simulink model "final4dof"  (R2016b)
settings: Solver=VariableStepAuto  StartTime=0.0  StopTime=inf  RelTol=1e-3
StartFcn:
  | 1
values from neighbouring files (symbols this model uses):
  N = sqrt(1-M*M)    [GUI_TA.m]
undefined symbols (not defined in the file or in its folder): final4dof, RootGround, RootPart
libraries: mblibv1 x18, simulink x4
settings Model: Creator=IMA F  LastModifiedBy=MILZAM_WAFI
settings OptimizationCC: BlockReduction=off
settings SimMechanicsCC: VisOnUpdateDiagram=on  VisDuringSimulation=on

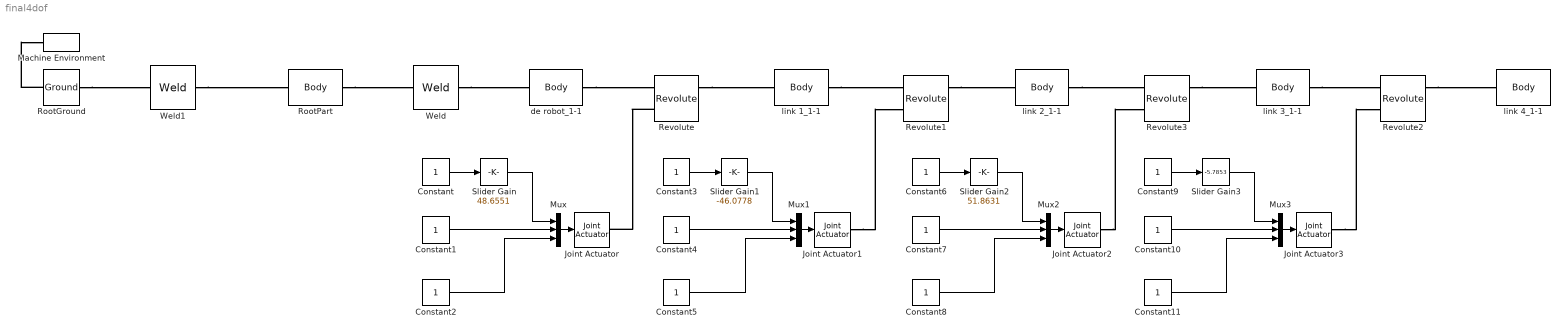
== system final4dof ==
  Constant{,1..11} (12 alike) : Constant
  Joint Actuator{,1..3} (4 alike) : mblibv1/Sensors &  Actuators/Joint Actuator  UpdateFromCAD=off  PhysicalDomain=Mechanical  PortType=blob  ActuationStyle=Motion  AngleUnits=deg  ArcVelocityUnits=deg/s  ArcAccelerationUnits=deg/s^2  CoordPositionUnits=m  VelocityUnits=m/s  AccelerationUnits=m/s^2  ForceUnits=N  TorqueUnits=N*m  ActiveIO=on  Width=3  DialogClass=MechanicalActuatorBlock  Primitive=R1  ReferenceFrame=Absolute (World)
  Machine Environment : mblibv1/Bodies/Machine Environment  PortType=env  PhysicalDomain=Mechanical  DialogTemplateClass=MECH.MachineEnvironment  SyncWhenCopied=off  Gravity=[0 -9.81 0]  GravityUnits=m/s^2  GravityAsSignal=off  Dimensionality=Auto-detect  AnalysisType=Forward dynamics  LinearAssemblyTolerance=1e-3  LinearAssemblyToleranceUnits=m  AngularAssemblyTolerance=1e-3  AngularAssemblyToleranceUnits=rad  ConstraintSolverType=Stabilizing  ConstraintRelTolerance=1e-4  ConstraintAbsTolerance=1e-4  UseRobustSingularityHandling=off  RedundancyAnalysisToleranceType=Automatically select tolerance  RedundancyAnalysisTolerance=1e-14  StatePerturbationType=Fixed  PerturbationSize=1e-5  VisualizeMachine=on  BodyVisualizationType=Use model default body geometries  BodyColorSelMode=Use model default  DefaultBodyColor=[1 0 0]
  Mux{,1..3} (4 alike) : Mux  Inputs=3
  Revolute : mblibv1/Joints/Revolute  LConnTagsString=__newl0|SA1  RConnTagsString=__newr0|SA1  UpdateFromCAD=on  PMImportedID=de robot_1-1:-:link 1_1-1  NumSAPorts=2  CutJoint=off  MarkAsCut=off  Primitives=prismatic  PrimitiveProps=R1$World$[0,0,-1]$revolute  DialogClass=JointBlock  R1Axis=[0,0,-1]
  Revolute1 : mblibv1/Joints/Revolute  LConnTagsString=__newl0|SA1  RConnTagsString=__newr0|SA1  UpdateFromCAD=on  PMImportedID=link 1_1-1:-:link 2_1-1  NumSAPorts=2  CutJoint=off  MarkAsCut=off  Primitives=prismatic  PrimitiveProps=R1$World$[-0.659109,-0.752048,0]$revolute  DialogClass=JointBlock  R1Axis=[-0.659109,-0.752048,0]
  Revolute2 : mblibv1/Joints/Revolute  LConnTagsString=__newl0|SA1  RConnTagsString=__newr0|SA1  UpdateFromCAD=on  PMImportedID=link 3_1-1:-:link 4_1-1  NumSAPorts=2  CutJoint=off  MarkAsCut=off  Primitives=prismatic  PrimitiveProps=R1$World$[-0.659109,-0.752048,0]$revolute  DialogClass=JointBlock  R1Axis=[-0.659109,-0.752048,0]
  Revolute3 : mblibv1/Joints/Revolute  LConnTagsString=__newl0|SA1  RConnTagsString=__newr0|SA1  UpdateFromCAD=on  PMImportedID=link 2_1-1:-:link 3_1-1  NumSAPorts=2  CutJoint=off  MarkAsCut=off  Primitives=prismatic  PrimitiveProps=R1$World$[-0.659109,-0.752048,0]$revolute  DialogClass=JointBlock  R1Axis=[-0.659109,-0.752048,0]
  RootGround : mblibv1/Bodies/Ground  UpdateFromCAD=on  PMImportedID=RootGround  LeftPortType=env  RightPortType=workingframe  PhysicalDomain=Mechanical  DialogClass=GroundBlock  CoordPosition=[0.12262,-0.0751039,0.137158]  CoordPositionUnits=m  StateVectorMgrId=0  MachineId=[1 0]  ShowEnvPort=on  ParameterChecksum=[2340468738, 1246277301, 2344666585, 387744393]  TopologyChecksum=[2589014121, 3397118713, 2794257843, 4184611350]
  RootPart : mblibv1/Bodies/Body  LConnTagsString=CS3  RConnTagsString=CS2  UpdateFromCAD=on  PMImportedID=final4dof/RootPart  DialogClass=MechanicalBodyBlock  Mass=0  MassUnits=kg  InertiaUnits=kg*m^2  Inertia=[0,0,0;0,0,0;0,0,0]  Shape=Cylinder  ShapeDims=[1 1]  ShapeUnits=m  ShapeUse=false  Density=1  DensityUnits=kg/m^3  DensityUse=false  GraphicsMode=MACHINE_DEFAULT  BodyColorSelMode=MACHINE_DEFAULT  BodyColor=[1;0;0]  AttachedToCS=CS1  CG=Right$CG$[0.12262 -0.0751039 0.137158]$WORLD$WORLD$m$[1 0 0;0 1 0;0 0 1]$3x3 Transform$rad$WORLD$false$final4dof/RootPart::CG(AUTOGEN)  WorkingFrames=Right$CS1$[0 0 0]$WORLD$WORLD$m$[1 0 0;0 1 0;0 0 1]$3x3 Transform$rad$WORLD$false$final4dof/RootPart::CS1(AUTOGEN)#Right$CS2$[0.136056 -0.0768268 0.0803688]$WORLD$WORLD$m$[1 0 0;0 1 0;0 0 1]$3x3 Transform$rad$WORLD$true$de robot_1-1:-:final4dof/RootPart::final4dof/RootPart(AUTOGEN)#Left$CS3$[0.12262 -0.0751039 0.137158]$WORLD$WORLD$m$[1 0 0;0 1 0;0 0 1]$3x3 Transform$rad$WORLD$true$RootGround:-:final4dof/RootPart::final4dof/RootPart(AUTOGEN)  CGPos=[0.12262 -0.0751039 0.137158]  CGRot=[1 0 0;0 1 0;0 0 1]  CS0Pos=[]  CS0Rot=[]  CS1Pos=[0 0 0]  CS1Rot=[1 0 0;0 1 0;0 0 1]  CS2Pos=[0.136056 -0.0768268 0.0803688]  CS2Rot=[1 0 0;0 1 0;0 0 1]  CS3Pos=[0.12262 -0.0751039 0.137158]  CS3Rot=[1 0 0;0 1 0;0 0 1]  CS4Pos=[]  CS4Rot=[]  CS5Pos=[]  CS5Rot=[]  CS6Pos=[]  CS6Rot=[]  CS7Pos=[]  CS7Rot=[]  CS8Pos=[]  CS8Rot=[]  CS9Pos=[]  CS9Rot=[]  CS10Pos=[]  CS10Rot=[]  CS11Pos=[]  CS11Rot=[]  CS12Pos=[]  CS12Rot=[]  CS13Pos=[]  CS13Rot=[]  CS14Pos=[]  CS14Rot=[]  CS15Pos=[]  CS15Rot=[]  CS16Pos=[]  CS16Rot=[]  CS17Pos=[]  CS17Rot=[]  CS18Pos=[]  CS18Rot=[]  CS19Pos=[]  CS19Rot=[]  CS20Pos=[]  CS20Rot=[]
  Slider Gain : simulink/Math Operations/Slider Gain  low=-360  gain=48.6551  high=360
  Slider Gain1 : simulink/Math Operations/Slider Gain  low=-360  gain=-46.0778  high=360
  Slider Gain2 : simulink/Math Operations/Slider Gain  low=-360  gain=51.8631  high=360
  Slider Gain3 : simulink/Math Operations/Slider Gain  low=-360  gain=-5.7853  high=360
  Weld : mblibv1/Joints/Weld  LConnTagsString=__newl0  RConnTagsString=__newr0  UpdateFromCAD=on  PMImportedID=de robot_1-1:-:final4dof/RootPart  NumSAPorts=0  CutJoint=off  MarkAsCut=off  Primitives=weld  PrimitiveProps=W$WORLD$[0.57735,0.57735,0.57735]$weld  DialogClass=JointBlock  WAxis=[0.57735,0.57735,0.57735]
  Weld1 : mblibv1/Joints/Weld  LConnTagsString=__newl0  RConnTagsString=__newr0  UpdateFromCAD=on  PMImportedID=RootGround:-:final4dof/RootPart  NumSAPorts=0  CutJoint=off  MarkAsCut=off  Primitives=weld  PrimitiveProps=W$WORLD$[0.57735,0.57735,0.57735]$weld  DialogClass=JointBlock  WAxis=[0.57735,0.57735,0.57735]
  de robot_1-1 : mblibv1/Bodies/Body  LConnTagsString=CS2  RConnTagsString=CS3  UpdateFromCAD=on  PMImportedID=de robot_1-1  DialogClass=MechanicalBodyBlock  Mass=0.451279  MassUnits=kg  InertiaUnits=kg*m^2  Inertia=[0.000359034,1.00878e-05,4.29188e-05;1.00878e-05,0.000788173,6.73587e-07;4.29188e-05,6.73587e-07,0.000996356]  Shape=Cylinder  ShapeDims=[1 1]  ShapeUnits=m  ShapeUse=false  Density=1  DensityUnits=kg/m^3  DensityUse=false  GraphicsMode=GFXFILE  GraphicsFileName=final4dof - de robot_1-1.STL  BodyColorSelMode=COLORPALETTE  BodyColor=[0.792157;0.819608;0.933333]  AttachedToCS=CS1  CG=Right$CG$[0.136056 -0.0768268 0.0803688]$WORLD$WORLD$m$[1 0 0;0 1 0;0 0 1]$3x3 Transform$rad$WORLD$false$de robot_1-1::CG(AUTOGEN)  WorkingFrames=Right$CS1$[0.113404 -0.0765211 0.0604763]$WORLD$WORLD$m$[1 0 0;0 1 0;0 0 1]$3x3 Transform$rad$WORLD$false$de robot_1-1::CS1(AUTOGEN)#Left$CS2$[0.136056 -0.0768268 0.0803688]$WORLD$WORLD$m$[1 0 0;0 1 0;0 0 1]$3x3 Transform$rad$WORLD$true$de robot_1-1:-:final4dof/RootPart::de robot_1-1(AUTOGEN)#Right$CS3$[0.113404 -0.0765211 0.115476]$WORLD$WORLD$m$[1 0 0;0 1 0;0 0 1]$3x3 Transform$rad$WORLD$true$de robot_1-1:-:link 1_1-1::de robot_1-1(AUTOGEN)  CGPos=[0.136056 -0.0768268 0.0803688]  CGRot=[1 0 0;0 1 0;0 0 1]  CS0Pos=[]  CS0Rot=[]  CS1Pos=[0.113404 -0.0765211 0.0604763]  CS1Rot=[1 0 0;0 1 0;0 0 1]  CS2Pos=[0.136056 -0.0768268 0.0803688]  CS2Rot=[1 0 0;0 1 0;0 0 1]  CS3Pos=[0.113404 -0.0765211 0.115476]  CS3Rot=[1 0 0;0 1 0;0 0 1]  CS4Pos=[]  CS4Rot=[]  CS5Pos=[]  CS5Rot=[]  CS6Pos=[]  CS6Rot=[]  CS7Pos=[]  CS7Rot=[]  CS8Pos=[]  CS8Rot=[]  CS9Pos=[]  CS9Rot=[]  CS10Pos=[]  CS10Rot=[]  CS11Pos=[]  CS11Rot=[]  CS12Pos=[]  CS12Rot=[]  CS13Pos=[]  CS13Rot=[]  CS14Pos=[]  CS14Rot=[]  CS15Pos=[]  CS15Rot=[]  CS16Pos=[]  CS16Rot=[]  CS17Pos=[]  CS17Rot=[]  CS18Pos=[]  CS18Rot=[]  CS19Pos=[]  CS19Rot=[]  CS20Pos=[]  CS20Rot=[]
  link 1_1-1 : mblibv1/Bodies/Body  LConnTagsString=CS2  RConnTagsString=CS3  UpdateFromCAD=on  PMImportedID=link 1_1-1  DialogClass=MechanicalBodyBlock  Mass=0.299894  MassUnits=kg  InertiaUnits=kg*m^2  Inertia=[0.000464896,-0.000192935,-6.22905e-10;-0.000192935,0.000282386,-2.05321e-09;-6.22905e-10,-2.05321e-09,0.000584377]  Shape=Cylinder  ShapeDims=[1 1]  ShapeUnits=m  ShapeUse=false  Density=1  DensityUnits=kg/m^3  DensityUse=false  GraphicsMode=GFXFILE  GraphicsFileName=final4dof - link 1_1-1.STL  BodyColorSelMode=COLORPALETTE  BodyColor=[0.792157;0.819608;0.933333]  AttachedToCS=CS1  CG=Right$CG$[0.0984995 -0.0634578 0.156058]$WORLD$WORLD$m$[0.752048 0 0.659109;-0.659109 0 0.752048;0 -1 0]$3x3 Transform$rad$WORLD$false$link 1_1-1::CG(AUTOGEN)  WorkingFrames=Right$CS1$[0.0758016 -0.0435656 0.205476]$WORLD$WORLD$m$[0.752048 0 0.659109;-0.659109 0 0.752048;0 -1 0]$3x3 Transform$rad$WORLD$false$link 1_1-1::CS1(AUTOGEN)#Left$CS2$[0.113404 -0.0765211 0.115476]$WORLD$WORLD$m$[1 0 0;0 1 0;0 0 1]$3x3 Transform$rad$WORLD$true$de robot_1-1:-:link 1_1-1::link 1_1-1(AUTOGEN)#Right$CS3$[0.0833814 -0.0349171 0.205476]$WORLD$WORLD$m$[1 0 0;0 1 0;0 0 1]$3x3 Transform$rad$WORLD$true$link 1_1-1:-:link 2_1-1::link 1_1-1(AUTOGEN)  CGPos=[0.0984995 -0.0634578 0.156058]  CGRot=[0.752048 0 0.659109;-0.659109 0 0.752048;0 -1 0]  CS0Pos=[]  CS0Rot=[]  CS1Pos=[0.0758016 -0.0435656 0.205476]  CS1Rot=[0.752048 0 0.659109;-0.659109 0 0.752048;0 -1 0]  CS2Pos=[0.113404 -0.0765211 0.115476]  CS2Rot=[1 0 0;0 1 0;0 0 1]  CS3Pos=[0.0833814 -0.0349171 0.205476]  CS3Rot=[1 0 0;0 1 0;0 0 1]  CS4Pos=[]  CS4Rot=[]  CS5Pos=[]  CS5Rot=[]  CS6Pos=[]  CS6Rot=[]  CS7Pos=[]  CS7Rot=[]  CS8Pos=[]  CS8Rot=[]  CS9Pos=[]  CS9Rot=[]  CS10Pos=[]  CS10Rot=[]  CS11Pos=[]  CS11Rot=[]  CS12Pos=[]  CS12Rot=[]  CS13Pos=[]  CS13Rot=[]  CS14Pos=[]  CS14Rot=[]  CS15Pos=[]  CS15Rot=[]  CS16Pos=[]  CS16Rot=[]  CS17Pos=[]  CS17Rot=[]  CS18Pos=[]  CS18Rot=[]  CS19Pos=[]  CS19Rot=[]  CS20Pos=[]  CS20Rot=[]
  link 2_1-1 : mblibv1/Bodies/Body  LConnTagsString=CS2  RConnTagsString=CS3  UpdateFromCAD=on  PMImportedID=link 2_1-1  DialogClass=MechanicalBodyBlock  Mass=0.110064  MassUnits=kg  InertiaUnits=kg*m^2  Inertia=[2.18831e-05,-1.87351e-06,-9.9891e-13;-1.87351e-06,0.000106749,-1.32509e-10;-9.9891e-13,-1.32509e-10,0.000107667]  Shape=Cylinder  ShapeDims=[1 1]  ShapeUnits=m  ShapeUse=false  Density=1  DensityUnits=kg/m^3  DensityUse=false  GraphicsMode=GFXFILE  GraphicsFileName=final4dof - link 2_1-1.STL  BodyColorSelMode=COLORPALETTE  BodyColor=[0.792157;0.819608;0.933333]  AttachedToCS=CS1  CG=Right$CG$[0.101292 -0.0659057 0.227905]$WORLD$WORLD$m$[0.617862 0.428746 0.659109;-0.541505 -0.375761 0.752048;0.570104 -0.821572 0]$3x3 Transform$rad$WORLD$false$link 2_1-1::CG(AUTOGEN)  WorkingFrames=Right$CS1$[0.132247 -0.0930353 0.255142]$WORLD$WORLD$m$[0.617862 0.428746 0.659109;-0.541505 -0.375761 0.752048;0.570104 -0.821572 0]$3x3 Transform$rad$WORLD$false$link 2_1-1::CS1(AUTOGEN)#Left$CS2$[0.0833814 -0.0349171 0.205476]$WORLD$WORLD$m$[1 0 0;0 1 0;0 0 1]$3x3 Transform$rad$WORLD$true$link 1_1-1:-:link 2_1-1::link 2_1-1(AUTOGEN)#Right$CS3$[0.151031 -0.0716019 0.255142]$WORLD$WORLD$m$[1 0 0;0 1 0;0 0 1]$3x3 Transform$rad$WORLD$true$link 2_1-1:-:link 3_1-1::link 2_1-1(AUTOGEN)  CGPos=[0.101292 -0.0659057 0.227905]  CGRot=[0.617862 0.428746 0.659109;-0.541505 -0.375761 0.752048;0.570104 -0.821572 0]  CS0Pos=[]  CS0Rot=[]  CS1Pos=[0.132247 -0.0930353 0.255142]  CS1Rot=[0.617862 0.428746 0.659109;-0.541505 -0.375761 0.752048;0.570104 -0.821572 0]  CS2Pos=[0.0833814 -0.0349171 0.205476]  CS2Rot=[1 0 0;0 1 0;0 0 1]  CS3Pos=[0.151031 -0.0716019 0.255142]  CS3Rot=[1 0 0;0 1 0;0 0 1]  CS4Pos=[]  CS4Rot=[]  CS5Pos=[]  CS5Rot=[]  CS6Pos=[]  CS6Rot=[]  CS7Pos=[]  CS7Rot=[]  CS8Pos=[]  CS8Rot=[]  CS9Pos=[]  CS9Rot=[]  CS10Pos=[]  CS10Rot=[]  CS11Pos=[]  CS11Rot=[]  CS12Pos=[]  CS12Rot=[]  CS13Pos=[]  CS13Rot=[]  CS14Pos=[]  CS14Rot=[]  CS15Pos=[]  CS15Rot=[]  CS16Pos=[]  CS16Rot=[]  CS17Pos=[]  CS17Rot=[]  CS18Pos=[]  CS18Rot=[]  CS19Pos=[]  CS19Rot=[]  CS20Pos=[]  CS20Rot=[]
  link 3_1-1 : mblibv1/Bodies/Body  LConnTagsString=CS3  RConnTagsString=CS2  UpdateFromCAD=on  PMImportedID=link 3_1-1  DialogClass=MechanicalBodyBlock  Mass=0.0552346  MassUnits=kg  InertiaUnits=kg*m^2  Inertia=[7.24126e-06,6.68018e-13,-8.04531e-13;6.68018e-13,6.73712e-05,7.87798e-12;-8.04531e-13,7.87798e-12,6.37418e-05]  Shape=Cylinder  ShapeDims=[1 1]  ShapeUnits=m  ShapeUse=false  Density=1  DensityUnits=kg/m^3  DensityUse=false  GraphicsMode=GFXFILE  GraphicsFileName=final4dof - link 3_1-1.STL  BodyColorSelMode=COLORPALETTE  BodyColor=[0.792157;0.819608;0.933333]  AttachedToCS=CS1  CG=Right$CG$[0.164509 -0.121311 0.280044]$WORLD$WORLD$m$[0.650411 0.377547 0.659109;-0.570032 -0.330889 0.752048;0.502025 -0.864853 0]$3x3 Transform$rad$WORLD$false$link 3_1-1::CG(AUTOGEN)  WorkingFrames=Right$CS1$[0.202491 -0.154599 0.309361]$WORLD$WORLD$m$[0.650411 0.377547 0.659109;-0.570032 -0.330889 0.752048;0.502025 -0.864853 0]$3x3 Transform$rad$WORLD$false$link 3_1-1::CS1(AUTOGEN)#Right$CS2$[0.206446 -0.150086 0.309361]$WORLD$WORLD$m$[1 0 0;0 1 0;0 0 1]$3x3 Transform$rad$WORLD$true$link 3_1-1:-:link 4_1-1::link 3_1-1(AUTOGEN)#Left$CS3$[0.151031 -0.0716019 0.255142]$WORLD$WORLD$m$[1 0 0;0 1 0;0 0 1]$3x3 Transform$rad$WORLD$true$link 2_1-1:-:link 3_1-1::link 3_1-1(AUTOGEN)  CGPos=[0.164509 -0.121311 0.280044]  CGRot=[0.650411 0.377547 0.659109;-0.570032 -0.330889 0.752048;0.502025 -0.864853 0]  CS0Pos=[]  CS0Rot=[]  CS1Pos=[0.202491 -0.154599 0.309361]  CS1Rot=[0.650411 0.377547 0.659109;-0.570032 -0.330889 0.752048;0.502025 -0.864853 0]  CS2Pos=[0.206446 -0.150086 0.309361]  CS2Rot=[1 0 0;0 1 0;0 0 1]  CS3Pos=[0.151031 -0.0716019 0.255142]  CS3Rot=[1 0 0;0 1 0;0 0 1]  CS4Pos=[]  CS4Rot=[]  CS5Pos=[]  CS5Rot=[]  CS6Pos=[]  CS6Rot=[]  CS7Pos=[]  CS7Rot=[]  CS8Pos=[]  CS8Rot=[]  CS9Pos=[]  CS9Rot=[]  CS10Pos=[]  CS10Rot=[]  CS11Pos=[]  CS11Rot=[]  CS12Pos=[]  CS12Rot=[]  CS13Pos=[]  CS13Rot=[]  CS14Pos=[]  CS14Rot=[]  CS15Pos=[]  CS15Rot=[]  CS16Pos=[]  CS16Rot=[]  CS17Pos=[]  CS17Rot=[]  CS18Pos=[]  CS18Rot=[]  CS19Pos=[]  CS19Rot=[]  CS20Pos=[]  CS20Rot=[]
  link 4_1-1 : mblibv1/Bodies/Body  LConnTagsString=CS2  UpdateFromCAD=on  PMImportedID=link 4_1-1  DialogClass=MechanicalBodyBlock  Mass=0.0126155  MassUnits=kg  InertiaUnits=kg*m^2  Inertia=[6.55182e-07,1.94579e-14,0;1.94579e-14,2.2097e-06,1.5085e-12;0,1.5085e-12,2.21192e-06]  Shape=Cylinder  ShapeDims=[1 1]  ShapeUnits=m  ShapeUse=false  Density=1  DensityUnits=kg/m^3  DensityUse=false  GraphicsMode=GFXFILE  GraphicsFileName=final4dof - link 4_1-1.STL  BodyColorSelMode=COLORPALETTE  BodyColor=[0.792157;0.819608;0.933333]  AttachedToCS=CS1  CG=Right$CG$[0.218034 -0.168262 0.302011]$WORLD$WORLD$m$[0.708681 -0.251688 0.659109;-0.621101 0.220584 0.752048;-0.33467 -0.942335 0]$3x3 Transform$rad$WORLD$false$link 4_1-1::CG(AUTOGEN)  WorkingFrames=Right$CS1$[0.246763 -0.193441 0.288444]$WORLD$WORLD$m$[0.708681 -0.251688 0.659109;-0.621101 0.220584 0.752048;-0.33467 -0.942335 0]$3x3 Transform$rad$WORLD$false$link 4_1-1::CS1(AUTOGEN)#Left$CS2$[0.206446 -0.150086 0.309361]$WORLD$WORLD$m$[1 0 0;0 1 0;0 0 1]$3x3 Transform$rad$WORLD$true$link 3_1-1:-:link 4_1-1::link 4_1-1(AUTOGEN)  CGPos=[0.218034 -0.168262 0.302011]  CGRot=[0.708681 -0.251688 0.659109;-0.621101 0.220584 0.752048;-0.33467 -0.942335 0]  CS0Pos=[]  CS0Rot=[]  CS1Pos=[0.246763 -0.193441 0.288444]  CS1Rot=[0.708681 -0.251688 0.659109;-0.621101 0.220584 0.752048;-0.33467 -0.942335 0]  CS2Pos=[0.206446 -0.150086 0.309361]  CS2Rot=[1 0 0;0 1 0;0 0 1]  CS3Pos=[]  CS3Rot=[]  CS4Pos=[]  CS4Rot=[]  CS5Pos=[]  CS5Rot=[]  CS6Pos=[]  CS6Rot=[]  CS7Pos=[]  CS7Rot=[]  CS8Pos=[]  CS8Rot=[]  CS9Pos=[]  CS9Rot=[]  CS10Pos=[]  CS10Rot=[]  CS11Pos=[]  CS11Rot=[]  CS12Pos=[]  CS12Rot=[]  CS13Pos=[]  CS13Rot=[]  CS14Pos=[]  CS14Rot=[]  CS15Pos=[]  CS15Rot=[]  CS16Pos=[]  CS16Rot=[]  CS17Pos=[]  CS17Rot=[]  CS18Pos=[]  CS18Rot=[]  CS19Pos=[]  CS19Rot=[]  CS20Pos=[]  CS20Rot=[]
  wires:
  Slider Gain/1 -> Mux/1
  Constant/1 -> Slider Gain/1
  Constant1/1 -> Mux/2
  Constant2/1 -> Mux/3
  Mux/1 -> Joint Actuator/1
  Slider Gain1/1 -> Mux1/1
  Constant3/1 -> Slider Gain1/1
  Constant4/1 -> Mux1/2
  Constant5/1 -> Mux1/3
  Mux1/1 -> Joint Actuator1/1
  Slider Gain2/1 -> Mux2/1
  Constant6/1 -> Slider Gain2/1
  Constant7/1 -> Mux2/2
  Constant8/1 -> Mux2/3
  Mux2/1 -> Joint Actuator2/1
  Slider Gain3/1 -> Mux3/1
  Constant9/1 -> Slider Gain3/1
  Constant10/1 -> Mux3/2
  Constant11/1 -> Mux3/3
  Mux3/1 -> Joint Actuator3/1
  connections:
  RootPart/RConn1 -- Weld/LConn1
  Weld/RConn1 -- de robot_1-1/LConn1
  de robot_1-1/RConn1 -- Revolute/LConn1
  Revolute/RConn1 -- link 1_1-1/LConn1
  link 1_1-1/RConn1 -- Revolute1/LConn1
  Revolute1/RConn1 -- link 2_1-1/LConn1
  link 3_1-1/RConn1 -- Revolute2/LConn1
  Revolute2/RConn1 -- link 4_1-1/LConn1
  link 2_1-1/RConn1 -- Revolute3/LConn1
  Revolute3/RConn1 -- link 3_1-1/LConn1
  RootGround/RConn1 -- Weld1/LConn1
  Weld1/RConn1 -- RootPart/LConn1
  RootGround/LConn1 -- Machine Environment/RConn1
  Revolute/LConn2 -- Joint Actuator/RConn1
  Joint Actuator1/RConn1 -- Revolute1/LConn2
  Joint Actuator2/RConn1 -- Revolute3/LConn2
  Joint Actuator3/RConn1 -- Revolute2/LConn2
